simulink model "daohang_2017b"  (R2017b)
settings: Solver=FixedStepAuto  StartTime=0.0  StopTime=80  FixedStep=0.01  MaxStep=0.01  RelTol=1e-3
undefined symbols (not defined in the file or in its folder): Earth, ini, Newton, Raphson, WGS84
libraries: sharedutil x2, sharedtransform x2, simulink_extras x2, shared6dof x1, aerolibatmos2 x1, aerolibobsolete x1, aerolibtransform2 x1
(part 2 of 2)

== system daohang_2017b/偏差/add noise3/Subsystem2/Markov process ==
  Add12 : Sum
  Gain : Gain  Gain=-1/ini.M_V_T
  Integrator : Integrator
  Memory11 : Memory
  Random Number13 : RandomNumber  Variance=ini.M_V_Variance  Seed=46  SampleTime=0.01
  Markov noise : Outport
  wires:
  Memory11/1 -> Gain/1
  Gain/1 -> Integrator/1
  Add12/1 -> Markov noise/1, Memory11/1
  Integrator/1 -> Add12/1
  Random Number13/1 -> Add12/2

== matlab function daohang_2017b/KF/FS ==
  data: FS output; cbn input
function FS = FS_build(cbn)
%FS = zeros(9,6);
temp = [0,-1,0;...
    -1,0,0;...
    0,0,-1;]*cbn;
temp = temp';
O33 = zeros(3,3);
FS = [O33,temp;...
    temp,O33;...
    O33,O33;];
end

== matlab function daohang_2017b/KF/FN  ==
  data: La input; FN output; g0 input; RN input; RM input; h input; vx input; vy input; vz input; fx input; fy input; fz input; omegaie input
function FN = FN_build(La,g0,RN,RM,h,vx,vy,vz,fx,fy,fz,omegaie)
FN = zeros(9,9);
tanl = tan(La);
sinl = sin(La);
cosl = cos(La);
Rnh = RN + h;
Rmh = RM + h;
FN(1,1) = (vy * tanl - vz)/Rnh;
FN(1,2) = 2*omegaie*sinl + vx*tanl/Rnh;
FN(1,3) = -(2*omegaie*cosl + vx/Rnh);
FN(1,5) = -fz;
FN(1,6) = fy;
FN(1,7) = (2*omegaie*vz*sinl+2*omegaie *vy*cosl+vx*vy/cosl/cosl/Rnh);
FN(2,1) = -(2*vx * tanl/Rnh + 2*omegaie *sinl);
FN(2,2) = -vz/Rmh;
FN(2,3) = -vy/Rmh;
FN(2,4) = -vz/Rmh;
FN(2,6) = -fx;
FN(2,7) = -(2*omegaie*cosl + vx/cosl/cosl/Rnh)*vx;
FN(3,1) = (2*omegaie*cosl + 2*vx/Rnh);
FN(3,2) = 2*vy/Rmh;
FN(3,4) = -fy;
FN(3,5) = fx;
FN(3,7) = -2*omegaie*vx*sinl;
FN(3,9) = 2*g0/RM;
FN(4,2) = -1/Rmh;
FN(4,5) = omegaie*sinl + vx/Rnh*tanl;
FN(4,6) = -omegaie *cosl -vx/Rnh;
FN(5,1) = 1/Rnh;
FN(5,4) = -omegaie *sinl -vx*tanl/Rnh;
FN(5,6) = -vy/Rmh;
FN(5,7) = -omegaie *sinl;
FN(6,1) = tanl/Rnh;
FN(6,4) = omegaie * cosl+vx/Rnh;
FN(6,5) = vy/Rmh;
FN(6,7) = omegaie*cosl + vx/cosl/cosl/Rnh;
FN(7,2) = 1/Rmh;
FN(8,1) = 1/cosl/Rnh;
FN(8,7) = vx/Rnh/cosl*tanl;
FN(9,3) =1;



end

== matlab function daohang_2017b/KF/FM ==
  data: tgx input; FM output; tgy input; tgz input; tax input; tay input; taz input
function FM = FM_build(tgx,tgy,tgz,tax,tay,taz)
FM = diag([-1/tgx,-1/tgy,-1/tgz,-1/tax,-1/tay,-1/taz]);
end

== matlab function daohang_2017b/KF/FI ==
  data: FN input; FI output; FS input; FM input
function FI= FI_build(FN,FS,FM)
FI = [FN,FS;zeros(6,9),FM];
end

== matlab function daohang_2017b/KF/MATLAB Function1 ==
  data: F input; PHI output; T input
function PHI = PHI_build(F,T)
PHI = eye(15,15)+T*F+T^2/4*F*F;
end

== matlab function daohang_2017b/KF/观测量 ==
  data: Rm input; Rn input; H output; Vn input; La input; Lo input; h input; VG input; Z output; PG input
function [H,Z]= ZH_build(Rm,Rn,Vn,La,Lo,h,VG,PG)
Z = zeros(6,1);
Zv=Vn-VG;
Zp=[(La-PG(1))*(Rm+h);
    (Lo-PG(2))*(Rn+h)*cos(La);
    h-PG(3)];
Z=[Zp;Zv];
%%%
H = zeros(6,15);
Hp=[zeros(3,6) diag([Rm+h;(Rn+h)*cos(La);1]) zeros(3,6)];
Hv=[diag([1;1;1]) zeros(3,12)];
H=[Hp;Hv];
end

== matlab function daohang_2017b/INS/MATLAB Function6 ==
  data: u input; y output
function y = fcn(u)
y = [u(1,1:3),u(2,1:3),u(3,1:3)];
end

== matlab function daohang_2017b/KF/MATLAB Function2 ==
  data: R output; g0 input; abai input; Q output; apiao input; omegabai input; omegapiao input
function [R,Q] = fcn(g0,abai,apiao,omegabai,omegapiao)
Q=zeros(15);
g = g0;
Q(1,1)=(abai*g)^2;
Q(2,2)=(abai*g)^2;
Q(3,3)=(abai*g)^2;
Q(4,4)=(omegabai/180*pi/3600)^2;
Q(5,5)=(omegabai/180*pi/3600)^2;
Q(6,6)=(omegabai/180*pi/3600)^2;
Q(10,10)=(omegapiao/180*pi/3600)^2;
Q(11,11)=(omegapiao/180*pi/3600)^2;
Q(12,12)=(omegapiao/180*pi/3600)^2;
Q(13,13)=(apiao*g)^2;
Q(14,14)=(apiao*g)^2;
Q(15,15)=(apiao*g)^2;
%Q = [8.46159499407524e-14,0,0,0,0,0,0,0,0,0,0,0,0,0,0;0,8.46159499407524e-14,0,0,0,0,0,0,0,0,0,0,0,0,0;0,0,8.46159499407524e-14,0,0,0,0,0,0,0,0,0,0,0,0;0,0,0,9.56484000000000e-11,0,0,0,0,0,0,0,0,0,0,0;0,0,0,0,9.56484000000000e-11,0,0,0,0,0,0,0,0,0,0;0,0,0,0,0,9.56484000000000e-11,0,0,0,0,0,0,0,0,0;0,0,0,0,0,0,0,0,0,0,0,0,0,0,0;0,0,0,0,0,0,0,0,0,0,0,0,0,0,0;0,0,0,0,0,0,0,0,0,0,0,0,0,0,0;0,0,0,0,0,0,0,0,0,0,0,0,0,0,0;0,0,0,0,0,0,0,0,0,0,0,0,0,0,0;0,0,0,0,0,0,0,0,0,0,0,0,0,0,0;0,0,0,0,0,0,0,0,0,0,0,0,0,0,0;0,0,0,0,0,0,0,0,0,0,0,0,0,0,0;0,0,0,0,0,0,0,0,0,0,0,0,0,0,0];
Re = 6378137; 
r = [[0.1;0.1;0.1];[[10;10]/Re;10]];  
R = diag(r)^2;
end

== matlab function daohang_2017b/KF/MATLAB Function ==
  data: u input; y output
function y = fcn(u)
y = u(1,1)+u(2,2)+u(3,3)+u(5,5)+u(4,4)+u(6,6)+u(7,7)+u(8,8)+u(9,9)+u(10,10)+u(11,11)+u(12,12)+u(13,13)+u(14,14)+u(15,15);
end

== matlab function daohang_2017b/KF/MATLAB Function3 ==
  data: R input; Xopt output; Q input; Xopt input; Popt input; PHi input; H input; Z input; Popt output; Vopt output; Laopt output; Loopt output; hopt output
function [Xopt,Popt,Vopt,Laopt,Loopt,hopt]= KF(R,Q,Xopt,Popt,PHi,H,Z)
Xpre=PHi*Xopt;            %15*1 = 15*15   *   15*1
Ppre=PHi*Popt*PHi'+Q;     %15*15   =   15*15   *  15*15   *    15*15  +  15*15
temp = H*Ppre*H';
if size(temp,1) == 6
    K=Ppre*H'*pinv(temp+R);    %15*6 =    15*15   *   15*6    /    (6*15 * 15*15 * 15*6 + 6*6)
    Xopt=Xpre+K*(Z-H*Xpre);   %15*1 = 15* 1 + 15*6  *  (6*1 - 6*15*15*1)
    Popt=(eye(15)-K*H)*Ppre*(eye(15)-K*H)'+K*R*K';     %15*15  =  (15*15 - 15*6  *  6*15) *  15*15  * (15*15 -  15*6 * 6*15) + 15*6 * 6*6 * 6*15
else
    K=Ppre*H'*pinv(temp);
    Xopt=Xpre+K*(Z-H*Xpre);   %15*1 = 15* 1 + 15*6  *  (6*1 - 6*15*15*1)
    Popt=(eye(15)-K*H)*Ppre*(eye(15)-K*H)';     %15*15  =  (15*15 - 15*6  *  6*15) *  15*15  * (15*15 -  15*6 * 6*15) + 15*6 * 6*6 * 6*15
end
Vopt = Xopt([1,2,3],1);
Laopt = Xopt(7,1);
Loopt = Xopt(8,1);
hopt = Xopt(9,1);
end

== matlab function daohang_2017b/INS/MATLAB Function10 ==
  data: g0 input; L input; g output
function g = g_cac(g0,L)

g=g0*(1+0.0052884*sin(L)*sin(L)-0.0000059*sin(2*L)*sin(2*L)); 
end

== matlab function daohang_2017b/INS/MATLAB Function11 ==
  data: u input; y output; h input; R input
function y = fcn(u, h,R)
y = u * (1-2*h/R);
end
